simulink model "P_Regler_Labor"  (R2018a)
settings: Solver=VariableStepAuto  StartTime=0.0  StopTime=0.4  RelTol=1e-3  EnableMultiTasking=on
values from neighbouring files (symbols this model uses):
  Cr = 7.2352*10^-6    (= 7.2352e-06)    [lab04_part01.m]    (also in lab05_part01_baga.m; lab06_simulationWithMeasurements.m)
  J = 5.5e-6    (= 5.5e-06)    [lab03_part01.m]    (also in lab04_part01.m = 8e-06; lab05_part01_baga.m = 8e-06; lab06_simulationWithMeasurements.m = 5.29e-06)
  ke = 0.017    [lab04_part01.m]    (also in lab05_part01_baga.m)
  km = 0.05    [lab04_part01.m]    (also in lab05_part01_baga.m)
  L = tan(phi).*Rges./(frequencies.*2*pi)    [lab02_part01.m]    (also in lab03_part01.m = 0.0005752; lab04_part01.m = 0.00035329; lab05_part01_baga.m = 0.00035329; lab06_simulationWithMeasurements.m = 0.000618)
  R_A = 3.22    [lab03_part01.m]    (also in lab05_part01_baga.m = 3.71; lab06_simulationWithMeasurements.m)
  R_S = 1    [lab03_part01.m]    (also in lab05_part01_baga.m; lab06_simulationWithMeasurements.m)
  w_soll = 450    [lab05_part01_baga.m]    (also in lab06_simulationWithMeasurements.m = 250)
undefined symbols (not defined in the file or in its folder): Tinterval
settings Model: Creator=Felix  LastModifiedBy=oleksandra
settings OptimizationCC: LifeSpan=inf
settings DebuggingCC: SFUnexpectedBacktrackingDiag=warning  SFNoUnconditionalDefaultTransitionDiag=warning  SFExecutionAtInitializationDiag=none
settings CodeAppCC: StateflowObjectComments=on
settings GRTTargetCC: TargetLangStandard=C89/C90 (ANSI)  GeneratePreprocessorConditionals=Disable all
settings ConfigComp: CovMetricSettings=dw  CovHtmlReporting=on  CovSaveCumulativeToWorkspaceVar=on  CovSaveSingleToWorkspaceVar=on  CovExternalEMLEnable=off

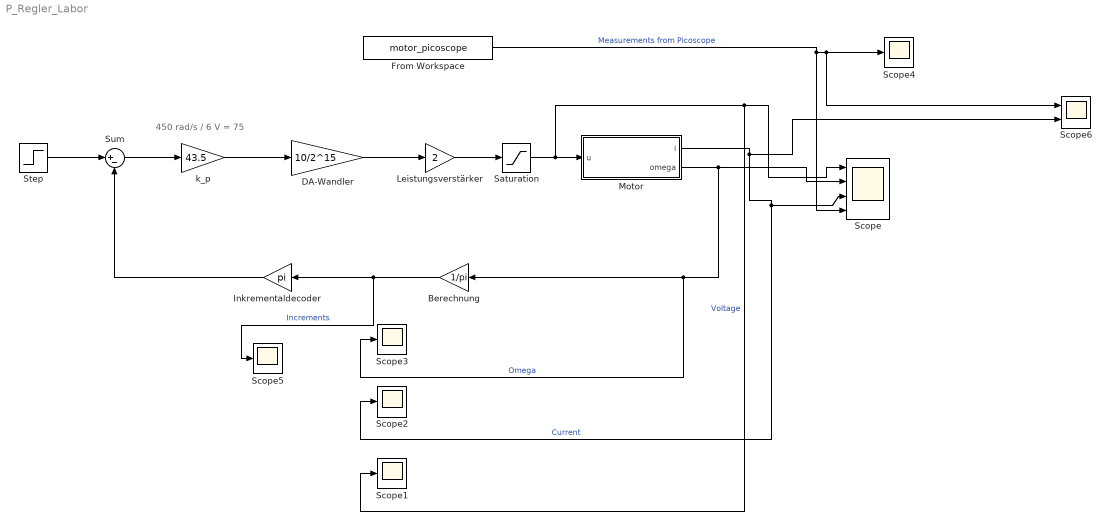
== system P_Regler_Labor ==
  note: 450 rad/s / 6 V = 75
  Berechnung : Gain  Gain=1/pi
  DA-Wandler : Gain  Gain=10/2^15
  From Workspace : FromWorkspace  VariableName=motor_picoscope  SampleTime=Tinterval
  Inkrementaldecoder : Gain  Gain=pi
  Leistungsverstärker : Gain  Gain=2
  Motor : Subsystem  TreatAsAtomicUnit=on
  Saturation : Saturate  UpperLimit=12  LowerLimit=-12
  Scope : Scope  NumInputPorts=4
  Scope{1..5} (5 alike) : Scope
  Scope6 : Scope  NumInputPorts=2
  Step : Step  Time=0.02  After=w_soll  SampleTime=0
  Sum : Sum  Inputs=|+-
  k_p : Gain  Gain=43.5
  wires:
  Leistungsverstärker/1 -> Saturation/1
  DA-Wandler/1 -> Leistungsverstärker/1
  k_p/1 -> DA-Wandler/1
  Sum/1 -> k_p/1
  Step/1 -> Sum/1
  Motor/2(omega) -> Scope3/1, Berechnung/1, Scope/2  "Omega"
  Motor/1(i) -> Scope6/2, Scope2/1, Scope/3  "Current"
  Saturation/1 -> Motor/1(u), Scope1/1, Scope/1  "Voltage"
  Berechnung/1 -> Scope5/1, Inkrementaldecoder/1  "Increments"
  Inkrementaldecoder/1 -> Sum/2
  From Workspace/1 -> Scope6/1, Scope4/1, Scope/4  "Measurements from Picoscope"

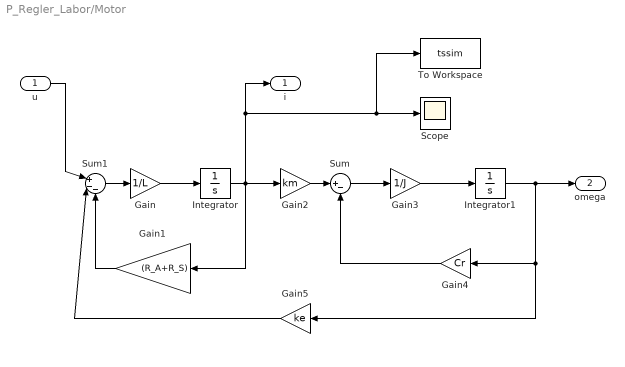
== system P_Regler_Labor/Motor ==
  u : Inport
  Gain : Gain  Gain=1/L  SaturateOnIntegerOverflow=on  OutDataTypeStr=Inherit: Same as input  ParamDataTypeStr=Inherit: Same as input
  Gain1 : Gain  Gain=(R_A+R_S)  SaturateOnIntegerOverflow=on  OutDataTypeStr=Inherit: Same as input  ParamDataTypeStr=Inherit: Same as input
  Gain2 : Gain  Gain=km  SaturateOnIntegerOverflow=on  OutDataTypeStr=Inherit: Same as input  ParamDataTypeStr=Inherit: Same as input
  Gain3 : Gain  Gain=1/J  SaturateOnIntegerOverflow=on  OutDataTypeStr=Inherit: Same as input  ParamDataTypeStr=Inherit: Same as input
  Gain4 : Gain  Gain=Cr  SaturateOnIntegerOverflow=on  OutDataTypeStr=Inherit: Same as input  ParamDataTypeStr=Inherit: Same as input
  Gain5 : Gain  Gain=ke  SaturateOnIntegerOverflow=on  OutDataTypeStr=Inherit: Same as input  ParamDataTypeStr=Inherit: Same as input
  Integrator : Integrator
  Integrator1 : Integrator
  Scope : Scope
  Sum : Sum  Inputs=|+-  SaturateOnIntegerOverflow=on  InputSameDT=on  OutDataTypeStr=Inherit: Same as first input
  Sum1 : Sum  Inputs=|+--  SaturateOnIntegerOverflow=on  InputSameDT=on  OutDataTypeStr=Inherit: Same as first input
  To Workspace : ToWorkspace  VariableName=tssim  SaveFormat=Timeseries  SampleTime=-1
  i : Outport  Unit=A
  omega : Outport  Port=2  Unit=1/s
  wires:
  Sum1/1 -> Gain/1
  Gain/1 -> Integrator/1
  Gain2/1 -> Sum/1
  Sum/1 -> Gain3/1
  Gain3/1 -> Integrator1/1
  Gain1/1 -> Sum1/3
  Gain4/1 -> Sum/2
  Integrator1/1 -> omega/1, Gain4/1, Gain5/1
  Gain5/1 -> Sum1/2
  Integrator/1 -> To Workspace/1, Scope/1, i/1, Gain2/1, Gain1/1
  u/1 -> Sum1/1
